simulink model "pend_ss_c"  (Simulink 5.0)
settings: Solver=ode45  StartTime=0.0  StopTime=10.0  RelTol=1e-3
values from neighbouring files (symbols this model uses):
  A = [-1 -2 0.5; 1 0 0; 0 1 0]    [ss_300.m]
  C = eye(4)    [pend.m]
  D = zeros(4,1)    [pend.m]
  K = P_/(P_+R)    [kal_ex.m]    (also in pend.m = place(a,b,P); ss_300.m = w(row,:))
  Ts = 0.01    [pend.m]
undefined symbols (not defined in the file or in its folder): B
settings Model: Creator=kannan  LastModifiedBy=kannan  ExtModeAutoUpdateStatusClock=off

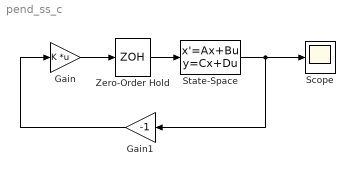
== system pend_ss_c ==
  Gain : Gain  Gain=K  Multiplication=Matrix(K*u)  SaturateOnIntegerOverflow=on
  Gain1 : Gain  Orientation=left  Gain=-1  SaturateOnIntegerOverflow=on
  Scope : Scope
  State-Space : StateSpace  A=A  B=B  C=C  D=D  X0=[0 0.1 0 0]
  Zero-Order Hold : ZeroOrderHold  SampleTime=Ts
  wires:
  State-Space/1 -> Scope/1, Gain1/1
  Gain/1 -> Zero-Order Hold/1
  Zero-Order Hold/1 -> State-Space/1
  Gain1/1 -> Gain/1
